simulink model "Noa_Nofusion_angle"  (R2020b)
settings: Solver=FixedStepDiscrete  StartTime=0.0  StopTime=Inf  FixedStep=0.01  RelTol=1e-3
PostLoadFcn:
  | if any(exist('dsrtsu_mdlpostloadfcn', 'file') ~= 0), dsrtsu_mdlpostloadfcn('Execute', bdroot); end
InitFcn:
  | , if any(exist('rtifpga_mdlclblib', 'file') ~= 0), rtifpga_mdlclblib('Init', bdroot); end,
  | , if any(exist('dsmpb_private', 'file') ~= 0), dsmpb_private('dsmpb_mdlclblib', 'Init', bdroot); end,
undefined symbols (not defined in the file): ACC_TimeGap_DecSetSwt, ACC_TimeGap_IncSetSwt, AccelPedalPosn, AccelPedalPosnVldty, AccelPedlPosnDiagc, AccPedalOverride, ACU_ShiftInProgress, ADAS_Posn_CurLane, AESSwtReq, ALC_SwtReq, BrkPedalSts, CC_ACC_CANCEL_OFFSwt, CC_ACC_CRUISE_OFFSwt, CC_ACC_DecSetSpd_SetSwt, CC_ACC_IncSetSpd_ResuSwt, CC_ACCSwtErr, CharSpd_ms, CSA_NODE, CURRENT_GEAR, CurrentGearValid, DiscIntNeverNeededParam, DrvDoorSts, DrvSBR, DrvTrqReqOvld, ECMACCInterface, ECMRespACC, ELKSwtReq, EngLimpHomeSts, EngSpd, EngState, EngState_PHEV, EngTrqMaxActSpd, EngTrqMinAct, EPS_DrvInpTrqVal_HighReslolution, EPS_FailSts, EPS_LKATorqOvrlDlvd, EPS_LKATorqOvrlDlvdVld, EPS_LKATrqOvlDlvdSts, EPS_SteerMod, EPS_TrqSnsrSts, EQ4_APPINFO, EQ4_LA_ELEM, EQ4_LA_HDR, EQ4_LAP_ELEM, EQ4_LAP_HDR, EQ4_LH_ELEM, EQ4_LH_HDR, EQ4_LRE_ELEM, EQ4_LRE_HDR, ESS_PedSwtReq, ESS_VehSwtReq, FFogLmpSts_F_Pbox, FLWheelDriveDirection, FLWheelSpd, FrntWiprSwtSts, FrntWshrSwtSts, FRWheelDriveDirection, FRWheelSpd, HazardLmpSwtSts, HCU_AccelPedalPosn_Diag ... (+151)
libraries: simulink x138, dsmpblib x33, canfdmsglib x10
(part 7 of 17)

== system Noa_Nofusion_angle/EQ4_Lane_Pack1/For Each Subsystem1 ==
  In1 : Inport  Partition=on  PartitionDimension=1  PartitionWidth=1  PartitionOffset=0
  Bus Assignment4 : BusAssignment  AssignedSignals=LH_CRC,LH_Is_Triggered_SDM_Type,LH_Is_Triggered_SDM_Model,LH_Track_ID,LH_Age,LH_Confidence,Reserved_3,LH_Prediction_Reason,LH_Availability_State,LH_Color,LH_Color_Confidence,LH_Lanemark_Type,LH_DLM_Type,LH_DECEL_Type,Reserved_4,LH_Lanemark_Type_Conf,LH_Side,LH_Crossing,LH_Marker_Width,LH_Marker_Width_STD,Reserved_5,LH_Dash_Average_Length,LH_Dash_Average_Gap,LH_Is_Multi_Clothoid,Reserved_6,LH_Line_First_C0,LH_Line_First_C1,LH_Line_First_C2,LH_Line_First_C3,LH_First_VR_Start,LH_First_VR_End,Reserved_7,LH_First_Measured_VR_End,LH_Second_Measured_VR_End,Reserved_8,LH_Line_Second_C0,LH_Line_Second_C1,LH_Line_Second_C2,LH_Line_Second_C3,LH_Second_VR_Start,LH_Second_VR_End,LH_Buffer_C3
  Bus Selector : BusSelector  OutputSignals=LH_CRC,LH_Is_Triggered_SDM_Type,LH_Is_Triggered_SDM_Model,LH_Track_ID,LH_Age,LH_Confidence,Reserved_3,LH_Prediction_Reason,LH_Availability_State,LH_Color,LH_Color_Confidence,LH_Lanemark_Type,LH_DLM_Type,LH_DECEL_Type,Reserved_4,LH_Lanemark_Type_Conf,LH_Side,LH_Crossing,LH_Marker_Width,LH_Marker_Width_STD,Reserved_5,LH_Dash_Average_Length,LH_Dash_Average_Gap,LH_Is_Multi_Clothoid,Reserved_6,LH_Line_First_C0,LH_Line_First_C1,LH_Line_First_C2,LH_Line_First_C3,LH_First_VR_Start,LH_First_VR_End,Reserved_7,LH_First_Measured_VR_End,LH_Second_Measured_VR_End,Reserved_8,LH_Line_Second_C0,LH_Line_Second_C1,LH_Line_Second_C2,LH_Line_Second_C3,LH_Second_VR_Start,LH_Second_VR_End,LH_Buffer_C3
  Constant4 : Constant  Value=0  OutDataTypeStr=Bus: EQ4_LH_ELEM_BUS
  For Each : ForEach  DisableCoverage=on
  Out1 : Outport  ConcatenationDimension=1
  wires:
  Constant4/1 -> Bus Assignment4/1
  In1/1 -> Bus Selector/1
  Bus Assignment4/1 -> Out1/1
  Bus Selector/1 -> Bus Assignment4/2  "<LH_CRC>"
  Bus Selector/2 -> Bus Assignment4/3  "<LH_Is_Triggered_SDM_Type>"
  Bus Selector/3 -> Bus Assignment4/4  "<LH_Is_Triggered_SDM_Model>"
  Bus Selector/4 -> Bus Assignment4/5  "<LH_Track_ID>"
  Bus Selector/5 -> Bus Assignment4/6  "<LH_Age>"
  Bus Selector/6 -> Bus Assignment4/7  "<LH_Confidence>"
  Bus Selector/7 -> Bus Assignment4/8  "<Reserved_3>"
  Bus Selector/8 -> Bus Assignment4/9  "<LH_Prediction_Reason>"
  Bus Selector/9 -> Bus Assignment4/10  "<LH_Availability_State>"
  Bus Selector/10 -> Bus Assignment4/11  "<LH_Color>"
  Bus Selector/11 -> Bus Assignment4/12  "<LH_Color_Confidence>"
  Bus Selector/12 -> Bus Assignment4/13  "<LH_Lanemark_Type>"
  Bus Selector/13 -> Bus Assignment4/14  "<LH_DLM_Type>"
  Bus Selector/14 -> Bus Assignment4/15  "<LH_DECEL_Type>"
  Bus Selector/15 -> Bus Assignment4/16  "<Reserved_4>"
  Bus Selector/16 -> Bus Assignment4/17  "<LH_Lanemark_Type_Conf>"
  Bus Selector/17 -> Bus Assignment4/18  "<LH_Side>"
  Bus Selector/18 -> Bus Assignment4/19  "<LH_Crossing>"
  Bus Selector/19 -> Bus Assignment4/20  "<LH_Marker_Width>"
  Bus Selector/20 -> Bus Assignment4/21  "<LH_Marker_Width_STD>"
  Bus Selector/21 -> Bus Assignment4/22  "<Reserved_5>"
  Bus Selector/22 -> Bus Assignment4/23  "<LH_Dash_Average_Length>"
  Bus Selector/23 -> Bus Assignment4/24  "<LH_Dash_Average_Gap>"
  Bus Selector/24 -> Bus Assignment4/25  "<LH_Is_Multi_Clothoid>"
  Bus Selector/25 -> Bus Assignment4/26  "<Reserved_6>"
  Bus Selector/26 -> Bus Assignment4/27  "<LH_Line_First_C0>"
  Bus Selector/27 -> Bus Assignment4/28  "<LH_Line_First_C1>"
  Bus Selector/28 -> Bus Assignment4/29  "<LH_Line_First_C2>"
  Bus Selector/29 -> Bus Assignment4/30  "<LH_Line_First_C3>"
  Bus Selector/30 -> Bus Assignment4/31  "<LH_First_VR_Start>"
  Bus Selector/31 -> Bus Assignment4/32  "<LH_First_VR_End>"
  Bus Selector/32 -> Bus Assignment4/33  "<Reserved_7>"
  Bus Selector/33 -> Bus Assignment4/34  "<LH_First_Measured_VR_End>"
  Bus Selector/34 -> Bus Assignment4/35  "<LH_Second_Measured_VR_End>"
  Bus Selector/35 -> Bus Assignment4/36  "<Reserved_8>"
  Bus Selector/36 -> Bus Assignment4/37  "<LH_Line_Second_C0>"
  Bus Selector/37 -> Bus Assignment4/38  "<LH_Line_Second_C1>"
  Bus Selector/38 -> Bus Assignment4/39  "<LH_Line_Second_C2>"
  Bus Selector/39 -> Bus Assignment4/40  "<LH_Line_Second_C3>"
  Bus Selector/40 -> Bus Assignment4/41  "<LH_Second_VR_Start>"
  Bus Selector/41 -> Bus Assignment4/42  "<LH_Second_VR_End>"
  Bus Selector/42 -> Bus Assignment4/43  "<LH_Buffer_C3>"

== system Noa_Nofusion_angle/EQ4_Lane_Pack1/For Each Subsystem2 ==
  In1 : Inport  Partition=on  PartitionDimension=1  PartitionWidth=1  PartitionOffset=0
  Bus Assignment4 : BusAssignment  AssignedSignals=LRE_ID,LRE_Age,LRE_Confidence,LRE_Type,Reserved_2,LRE_Prediction_Reason,LRE_Availability_State,LRE_Height,LRE_Height_STD,Reserved_3,LRE_View_Range_Start,LRE_View_Range_End,Reserved_4,LRE_Measured_VR_End,LRE_Side,LRE_Is_Triggered_SDM_Model,Reserved_5,LRE_Line_C3,LRE_Line_C2,LRE_Line_C1,LRE_Line_C0,LRE_Detection_Source,Reserved_6
  Bus Selector : BusSelector  OutputSignals=LRE_ID,LRE_Age,LRE_Confidence,LRE_Type,Reserved_2,LRE_Prediction_Reason,LRE_Availability_State,LRE_Height,LRE_Height_STD,Reserved_3,LRE_View_Range_Start,LRE_View_Range_End,Reserved_4,LRE_Measured_VR_End,LRE_Side,LRE_Is_Triggered_SDM_Model,Reserved_5,LRE_Line_C3,LRE_Line_C2,LRE_Line_C1,LRE_Line_C0,LRE_Detection_Source,Reserved_6
  Constant4 : Constant  Value=0  OutDataTypeStr=Bus: EQ4_LRE_ELEM_BUS
  For Each : ForEach  DisableCoverage=on
  Out1 : Outport  ConcatenationDimension=1
  wires:
  Bus Assignment4/1 -> Out1/1
  In1/1 -> Bus Selector/1
  Constant4/1 -> Bus Assignment4/1
  Bus Selector/1 -> Bus Assignment4/2  "<LRE_ID>"
  Bus Selector/2 -> Bus Assignment4/3  "<LRE_Age>"
  Bus Selector/3 -> Bus Assignment4/4  "<LRE_Confidence>"
  Bus Selector/4 -> Bus Assignment4/5  "<LRE_Type>"
  Bus Selector/5 -> Bus Assignment4/6  "<Reserved_2>"
  Bus Selector/6 -> Bus Assignment4/7  "<LRE_Prediction_Reason>"
  Bus Selector/7 -> Bus Assignment4/8  "<LRE_Availability_State>"
  Bus Selector/8 -> Bus Assignment4/9  "<LRE_Height>"
  Bus Selector/9 -> Bus Assignment4/10  "<LRE_Height_STD>"
  Bus Selector/10 -> Bus Assignment4/11  "<Reserved_3>"
  Bus Selector/11 -> Bus Assignment4/12  "<LRE_View_Range_Start>"
  Bus Selector/12 -> Bus Assignment4/13  "<LRE_View_Range_End>"
  Bus Selector/13 -> Bus Assignment4/14  "<Reserved_4>"
  Bus Selector/14 -> Bus Assignment4/15  "<LRE_Measured_VR_End>"
  Bus Selector/15 -> Bus Assignment4/16  "<LRE_Side>"
  Bus Selector/16 -> Bus Assignment4/17  "<LRE_Is_Triggered_SDM_Model>"
  Bus Selector/17 -> Bus Assignment4/18  "<Reserved_5>"
  Bus Selector/18 -> Bus Assignment4/19  "<LRE_Line_C3>"
  Bus Selector/19 -> Bus Assignment4/20  "<LRE_Line_C2>"
  Bus Selector/20 -> Bus Assignment4/21  "<LRE_Line_C1>"
  Bus Selector/21 -> Bus Assignment4/22  "<LRE_Line_C0>"
  Bus Selector/22 -> Bus Assignment4/23  "<LRE_Detection_Source>"
  Bus Selector/23 -> Bus Assignment4/24  "<Reserved_6>"

== system Noa_Nofusion_angle/EQ4_Lane_Pack1/For Each Subsystem3 ==
  In1 : Inport  Partition=on  PartitionDimension=1  PartitionWidth=1  PartitionOffset=0
  Bus Assignment4 : BusAssignment  AssignedSignals=LA_Lane_Track_ID,LA_Age,LA_Confidence,LA_Color,LA_Color_Conf,LA_Prediction_Reason,LA_Availability_State,LA_View_Range_Start,Reserved_2,LA_View_Range_End,LA_Measured_VR_End,Reserved_3,LA_Lanemark_Type,LA_DLM_Type,LA_Lanemark_Type_Conf,LA_Line_Side,LA_Marker_Width,Reserved_4,LA_Marker_Width_STD,Reserved_5,LA_Line_C3,LA_Line_C2,LA_Line_C1,LA_Line_C0,LH_Buffer_C1,Reserved_6
  Bus Selector : BusSelector  OutputSignals=LA_Lane_Track_ID,LA_Age,LA_Confidence,LA_Color,LA_Color_Conf,LA_Prediction_Reason,LA_Availability_State,LA_View_Range_Start,Reserved_2,LA_View_Range_End,LA_Measured_VR_End,Reserved_3,LA_Lanemark_Type,LA_DLM_Type,LA_Lanemark_Type_Conf,LA_Line_Side,LA_Marker_Width,Reserved_4,LA_Marker_Width_STD,Reserved_5,LA_Line_C3,LA_Line_C2,LA_Line_C1,LA_Line_C0,LH_Buffer_C1,Reserved_6
  Constant4 : Constant  Value=0  OutDataTypeStr=Bus: EQ4_LA_ELEM_BUS
  For Each : ForEach  DisableCoverage=on
  Out1 : Outport  ConcatenationDimension=1
  wires:
  Bus Assignment4/1 -> Out1/1
  In1/1 -> Bus Selector/1
  Constant4/1 -> Bus Assignment4/1
  Bus Selector/1 -> Bus Assignment4/2  "<LA_Lane_Track_ID>"
  Bus Selector/2 -> Bus Assignment4/3  "<LA_Age>"
  Bus Selector/3 -> Bus Assignment4/4  "<LA_Confidence>"
  Bus Selector/4 -> Bus Assignment4/5  "<LA_Color>"
  Bus Selector/5 -> Bus Assignment4/6  "<LA_Color_Conf>"
  Bus Selector/6 -> Bus Assignment4/7  "<LA_Prediction_Reason>"
  Bus Selector/7 -> Bus Assignment4/8  "<LA_Availability_State>"
  Bus Selector/8 -> Bus Assignment4/9  "<LA_View_Range_Start>"
  Bus Selector/9 -> Bus Assignment4/10  "<Reserved_2>"
  Bus Selector/10 -> Bus Assignment4/11  "<LA_View_Range_End>"
  Bus Selector/11 -> Bus Assignment4/12  "<LA_Measured_VR_End>"
  Bus Selector/12 -> Bus Assignment4/13  "<Reserved_3>"
  Bus Selector/13 -> Bus Assignment4/14  "<LA_Lanemark_Type>"
  Bus Selector/14 -> Bus Assignment4/15  "<LA_DLM_Type>"
  Bus Selector/15 -> Bus Assignment4/16  "<LA_Lanemark_Type_Conf>"
  Bus Selector/16 -> Bus Assignment4/17  "<LA_Line_Side>"
  Bus Selector/17 -> Bus Assignment4/18  "<LA_Marker_Width>"
  Bus Selector/18 -> Bus Assignment4/19  "<Reserved_4>"
  Bus Selector/19 -> Bus Assignment4/20  "<LA_Marker_Width_STD>"
  Bus Selector/20 -> Bus Assignment4/21  "<Reserved_5>"
  Bus Selector/21 -> Bus Assignment4/22  "<LA_Line_C3>"
  Bus Selector/22 -> Bus Assignment4/23  "<LA_Line_C2>"
  Bus Selector/23 -> Bus Assignment4/24  "<LA_Line_C1>"
  Bus Selector/24 -> Bus Assignment4/25  "<LA_Line_C0>"
  Bus Selector/25 -> Bus Assignment4/26  "<LH_Buffer_C1>"
  Bus Selector/26 -> Bus Assignment4/27  "<Reserved_6>"

== system Noa_Nofusion_angle/EQ4_Lane_Pack1/For Each Subsystem4 ==
  In1 : Inport  Partition=on  PartitionDimension=1  PartitionWidth=1  PartitionOffset=0
  Bus Assignment4 : BusAssignment  AssignedSignals=LAP_INTP_ID,LAP_INTP_Distance_Age,LAP_INTP_Confidence,LAP_INTP_Is_Valid,LAP_INTP_Type,LAP_INTP_Is_Start,Reserved_4,LAP_INTP_Lat_Distance,LAP_INTP_Long_Distance,Reserved_5,LAP_Buffer_C1,LAP_Buffer_C2,Reserved_6
  Bus Selector : BusSelector  OutputSignals=LAP_INTP_ID,LAP_INTP_Distance_Age,LAP_INTP_Confidence,LAP_INTP_Is_Valid,LAP_INTP_Type,LAP_INTP_Is_Start,Reserved_4,LAP_INTP_Lat_Distance,LAP_INTP_Long_Distance,Reserved_5,LAP_Buffer_C1,LAP_Buffer_C2,Reserved_6,Reserved_7
  Constant4 : Constant  Value=0  OutDataTypeStr=Bus: EQ4_LAP_ELEM_BUS
  For Each : ForEach  DisableCoverage=on
  Out1 : Outport  ConcatenationDimension=1
  wires:
  Constant4/1 -> Bus Assignment4/1
  In1/1 -> Bus Selector/1
  Bus Assignment4/1 -> Out1/1
  Bus Selector/1 -> Bus Assignment4/2  "<LAP_INTP_ID>"
  Bus Selector/2 -> Bus Assignment4/3  "<LAP_INTP_Distance_Age>"
  Bus Selector/3 -> Bus Assignment4/4  "<LAP_INTP_Confidence>"
  Bus Selector/4 -> Bus Assignment4/5  "<LAP_INTP_Is_Valid>"
  Bus Selector/5 -> Bus Assignment4/6  "<LAP_INTP_Type>"
  Bus Selector/6 -> Bus Assignment4/7  "<LAP_INTP_Is_Start>"
  Bus Selector/7 -> Bus Assignment4/8  "<Reserved_4>"
  Bus Selector/8 -> Bus Assignment4/9  "<LAP_INTP_Lat_Distance>"
  Bus Selector/9 -> Bus Assignment4/10  "<LAP_INTP_Long_Distance>"
  Bus Selector/10 -> Bus Assignment4/11  "<Reserved_5>"
  Bus Selector/11 -> Bus Assignment4/12  "<LAP_Buffer_C1>"
  Bus Selector/12 -> Bus Assignment4/13  "<LAP_Buffer_C2>"
  Bus Selector/13 -> Bus Assignment4/14  "<Reserved_6>"

== system Noa_Nofusion_angle/LPV/ABM_Pack ==
  In1 : Inport
  Bus Assignment2 : BusAssignment  AssignedSignals=DrvSBR,PassSBR,VehLgtAccel,VehLatAccel,VehYawRate
  Bus Selector14 : BusSelector  OutputSignals=ABM_NODE.ABM1_MSG.DrvSBR,ABM_NODE.ABM1_MSG.PassSBR,ABM_NODE.ABM2_MSG.VehLgtAccel,ABM_NODE.ABM2_MSG.VehLatAccel,ABM_NODE.ABM2_MSG.VehYawRate
  Constant3 : Constant  Value=0  OutDataTypeStr=Bus: VCAN_ABM_MSG_BUS
  VSM_VCAN_ABM : Outport
  wires:
  Bus Assignment2/1 -> VSM_VCAN_ABM/1
  In1/1 -> Bus Selector14/1
  Constant3/1 -> Bus Assignment2/1
  Bus Selector14/5 -> Bus Assignment2/6  "<VehYawRate>"
  Bus Selector14/4 -> Bus Assignment2/5  "<VehLatAccel>"
  Bus Selector14/3 -> Bus Assignment2/4  "<VehLgtAccel>"
  Bus Selector14/2 -> Bus Assignment2/3  "<PassSBR>"
  Bus Selector14/1 -> Bus Assignment2/2  "<DrvSBR>"

== system Noa_Nofusion_angle/LPV/BCM_Pack ==
  In1 : Inport
  Bus Assignment2 : BusAssignment  AssignedSignals=WiprReq_F_PBOX,DrvDoorSts,PassengerDoorSts,WindshldWiprActvSts,HazardLmpSwtSts,KL30BRelaySts
  Bus Selector10 : BusSelector  OutputSignals=BCM_NODE.BCM8_MSG.WiprReq_F_PBOX,BCM_NODE.BCM1_MSG.DrvDoorSts,BCM_NODE.BCM1_MSG.PassengerDoorSts,BCM_NODE.BCM1_MSG.WindshldWiprActvSts,BCM_NODE.BCM3_MSG.HazardLmpSwtSts,BCM_NODE.BCM8_MSG.KL30BRelaySts
  Constant3 : Constant  Value=0  OutDataTypeStr=Bus: VCAN_BCM_MSG_BUS
  VSM_VCAN_BCM : Outport
  wires:
  In1/1 -> Bus Selector10/1
  Bus Assignment2/1 -> VSM_VCAN_BCM/1
  Constant3/1 -> Bus Assignment2/1
  Bus Selector10/3 -> Bus Assignment2/4  "<PassengerDoorSts>"
  Bus Selector10/4 -> Bus Assignment2/5  "<WindshldWiprActvSts>"
  Bus Selector10/2 -> Bus Assignment2/3  "<DrvDoorSts>"
  Bus Selector10/5 -> Bus Assignment2/6  "<HazardLmpSwtSts>"
  Bus Selector10/1 -> Bus Assignment2/2  "<WiprReq_F_PBOX>"
  Bus Selector10/6 -> Bus Assignment2/7  "<KL30BRelaySts>"

== system Noa_Nofusion_angle/LPV/CSA_Pack ==
  In1 : Inport
  Bus Assignment2 : BusAssignment  AssignedSignals=FrntWshrSwtSts,FrntWiprSwtSts,LTurnLmpSwtSts,RTurnLmpSwtSts,SteerWheelAng,SteerWheelAngSign,SteerWheelSpd,SteerWheelSpdSign,SAS_Sts,ACC_TimeGap_IncSetSwt,ACC_TimeGap_DecSetSwt,CC_ACC_CRUISE_OFFSwt,CC_ACC_CANCEL_OFFSwt,CC_ACC_IncSetSpd_ResuSwt,CC_ACC_DecSetSpd_SetSwt,CC_ACCSwtErr,HWA_OK_OFFSwt
  Bus Selector13 : BusSelector  OutputSignals=CSA_NODE.CSA1_MSG.FrntWshrSwtSts,CSA_NODE.CSA1_MSG.FrntWiprSwtSts,CSA_NODE.CSA1_MSG.LTurnLmpSwtSts,CSA_NODE.CSA1_MSG.RTurnLmpSwtSts,CSA_NODE.CSA2_MSG.SteerWheelAng,CSA_NODE.CSA2_MSG.SteerWheelAngSign,CSA_NODE.CSA2_MSG.SteerWheelSpd,CSA_NODE.CSA2_MSG.SteerWheelSpdSign,CSA_NODE.CSA2_MSG.SAS_Sts,CSA_NODE.CSA2_MSG.ACC_TimeGap_IncSetSwt,CSA_NODE.CSA2_MSG.ACC_TimeGap_DecSetSwt,CSA_NODE.CSA2_MSG.CC_ACC_CRUISE_OFFSwt,CSA_NODE.CSA2_MSG.CC_ACC_CANCEL_OFFSwt,CSA_NODE.CSA2_MSG.CC_ACC_IncSetSpd_ResuSwt,CSA_NODE.CSA2_MSG.CC_ACC_DecSetSpd_SetSwt,CSA_NODE.CSA2_MSG.CC_ACCSwtErr,CSA_NODE.CSA2_MSG.HWA_OK_OFFSwt
  Constant3 : Constant  Value=0  OutDataTypeStr=Bus: VCAN_CSA_MSG_BUS
  VSM_VCAN_CSA : Outport
  wires:
  In1/1 -> Bus Selector13/1
  Bus Assignment2/1 -> VSM_VCAN_CSA/1
  Constant3/1 -> Bus Assignment2/1
  Bus Selector13/1 -> Bus Assignment2/2  "<FrntWshrSwtSts>"
  Bus Selector13/2 -> Bus Assignment2/3  "<FrntWiprSwtSts>"
  Bus Selector13/3 -> Bus Assignment2/4  "<LTurnLmpSwtSts>"
  Bus Selector13/4 -> Bus Assignment2/5  "<RTurnLmpSwtSts>"
  Bus Selector13/5 -> Bus Assignment2/6  "<SteerWheelAng>"
  Bus Selector13/6 -> Bus Assignment2/7  "<SteerWheelAngSign>"
  Bus Selector13/7 -> Bus Assignment2/8  "<SteerWheelSpd>"
  Bus Selector13/8 -> Bus Assignment2/9  "<SteerWheelSpdSign>"
  Bus Selector13/9 -> Bus Assignment2/10  "<SAS_Sts>"
  Bus Selector13/10 -> Bus Assignment2/11  "<ACC_TimeGap_IncSetSwt>"
  Bus Selector13/11 -> Bus Assignment2/12  "<ACC_TimeGap_DecSetSwt>"
  Bus Selector13/12 -> Bus Assignment2/13  "<CC_ACC_CRUISE_OFFSwt>"
  Bus Selector13/13 -> Bus Assignment2/14  "<CC_ACC_CANCEL_OFFSwt>"
  Bus Selector13/14 -> Bus Assignment2/15  "<CC_ACC_IncSetSpd_ResuSwt>"
  Bus Selector13/15 -> Bus Assignment2/16  "<CC_ACC_DecSetSpd_SetSwt>"
  Bus Selector13/16 -> Bus Assignment2/17  "<CC_ACCSwtErr>"
  Bus Selector13/17 -> Bus Assignment2/18  "<HWA_OK_OFFSwt>"

== system Noa_Nofusion_angle/LPV/DCT_Pack ==
  In1 : Inport
  Bus Assignment : BusAssignment  AssignedSignals=CurrentGearValid,SHIFT_IN_PROGRESS,TargetGearValid,TARGET_GEAR,ShiftInPrgValid,CURRENT_GEAR,TGS_LEVER
  Bus Selector7 : BusSelector  OutputSignals=DCT_NODE.DCT5_MSG.CurrentGearValid,DCT_NODE.DCT5_MSG.SHIFT_IN_PROGRESS,DCT_NODE.DCT5_MSG.TargetGearValid,DCT_NODE.DCT5_MSG.TARGET_GEAR,DCT_NODE.DCT5_MSG.ShiftInPrgValid,DCT_NODE.DCT5_MSG.CURRENT_GEAR,DCT_NODE.DCT5_MSG.TGS_LEVER
  Constant1 : Constant  Value=0  OutDataTypeStr=Bus: VCAN_DCT_MSG_BUS
  VSM_VCAN_DCT : Outport
  wires:
  In1/1 -> Bus Selector7/1
  Constant1/1 -> Bus Assignment/1
  Bus Selector7/1 -> Bus Assignment/2  "<CurrentGearValid>"
  Bus Selector7/2 -> Bus Assignment/3  "<SHIFT_IN_PROGRESS>"
  Bus Selector7/3 -> Bus Assignment/4  "<TargetGearValid>"
  Bus Selector7/4 -> Bus Assignment/5  "<TARGET_GEAR>"
  Bus Selector7/5 -> Bus Assignment/6  "<ShiftInPrgValid>"
  Bus Selector7/6 -> Bus Assignment/7  "<CURRENT_GEAR>"
  Bus Selector7/7 -> Bus Assignment/8  "<TGS_LEVER>"
  Bus Assignment/1 -> VSM_VCAN_DCT/1

== system Noa_Nofusion_angle/LPV/ECM_Pack ==
  In1 : Inport
  Bus Assignment : BusAssignment  AssignedSignals=BrkPedalSts,EngSpd,Start_StopSts,AccPedalOverride,AccelPedlPosnDiagc,ECMRespACC,ECMACCInterface,AccelPedalPosn,AccelPedalPosnVldty,EngState,EngLimpHomeSts,EngState_PHEV
  Bus Selector6 : BusSelector  OutputSignals=ECM_NODE.ECM_FD1_MSG.BrkPedalSts,ECM_NODE.ECM_FD1_MSG.EngSpd,ECM_NODE.ECM_FD1_MSG.Start_StopSts,ECM_NODE.ECM_FD2_MSG.AccPedalOverride,ECM_NODE.ECM_FD2_MSG.AccelPedlPosnDiagc,ECM_NODE.ECM_FD2_MSG.ECMRespACC,ECM_NODE.ECM_FD2_MSG.ECMACCInterface,ECM_NODE.ECM_FD2_MSG.AccelPedalPosn,ECM_NODE.ECM_FD2_MSG.AccelPedalPosnVldty,ECM_NODE.ECM_FD2_MSG.EngState,ECM_NODE.ECM_FD3_MSG.EngLimpHomeSts
  Constant : Constant  Value=0x2
  Constant1 : Constant  Value=0  OutDataTypeStr=Bus: VCAN_ECM_MSG_BUS
  VSM_VCAN_ECM : Outport
  wires:
  In1/1 -> Bus Selector6/1
  Constant1/1 -> Bus Assignment/1
  Bus Assignment/1 -> VSM_VCAN_ECM/1
  Bus Selector6/5 -> Bus Assignment/6  "<AccelPedlPosnDiagc>"
  Bus Selector6/4 -> Bus Assignment/5  "<AccPedalOverride>"
  Bus Selector6/6 -> Bus Assignment/7  "<ECMRespACC>"
  Bus Selector6/3 -> Bus Assignment/4  "<Start_StopSts>"
  Bus Selector6/7 -> Bus Assignment/8  "<ECMACCInterface>"
  Bus Selector6/2 -> Bus Assignment/3  "<EngSpd>"
  Bus Selector6/8 -> Bus Assignment/9  "<AccelPedalPosn>"
  Bus Selector6/1 -> Bus Assignment/2  "<BrkPedalSts>"
  Bus Selector6/9 -> Bus Assignment/10  "<AccelPedalPosnVldty>"
  Bus Selector6/10 -> Bus Assignment/11  "<EngState>"
  Bus Selector6/11 -> Bus Assignment/12  "<EngLimpHomeSts>"
  Constant/1 -> Bus Assignment/13

== system Noa_Nofusion_angle/LPV/ESP_Pack ==
  In1 : Inport
  Bus Assignment : BusAssignment  AssignedSignals=BrkDskOvrheatd,NoBrkForce,VehStandstill,HDCCtrl,CDDActv,CDDAvailable,AVHSts,DrivingModDis,ESPFuncOffSts,ESPBrkLmpCtrl,ESPFailSts,ESP_MasterCylBrkPressVld,MSRActv,VDCActv,PTCActv,BTCActv,ESP_MasterCylBrkPress,MSRActv_RA,PTCActv_RA,BTCActv_RA,ABSFailSts,EBDFailSts,VehSpd,ABSActv,EPBSts,EPB_SwtPosn,RLWheelDriveDirection,RLWheelSpd,RRWheelDriveDirection,RRWheelSpd
  Bus Assignment1 : BusAssignment  AssignedSignals=EPS_FailSts,EPS_TrqSnsrSts,EPS_SteerMod,EPS_LKATorqOvrlDlvd,EPS_LKATorqOvrlDlvdVld,EPS_LKATrqOvlDlvdSts,EPS_DrvInpTrqVal_HighReslolution
  Bus Assignment2 : BusAssignment  AssignedSignals=SysPowerMod
  Bus Selector8 : BusSelector  OutputSignals=ESP_NODE.ESP_FD2_MSG.BrkDskOvrheatd,ESP_NODE.ESP_FD2_MSG.NoBrkForce,ESP_NODE.ESP_FD2_MSG.VehStandstill,ESP_NODE.ESP_FD2_MSG.HDCCtrl,ESP_NODE.ESP_FD2_MSG.CDDActv,ESP_NODE.ESP_FD2_MSG.CDDAvailable,ESP_NODE.ESP_FD2_MSG.AVHSts,ESP_NODE.ESP_FD2_MSG.DrivingModDis,ESP_NODE.ESP_FD2_MSG.ESPFuncOffSts,ESP_NODE.ESP_FD2_MSG.ESPBrkLmpCtrl,ESP_NODE.ESP_FD2_MSG.ESPFailSts,ESP_NODE.ESP_FD2_MSG.ESP_MasterCylBrkPressVld,ESP_NODE.ESP_FD2_MSG.MSRActv,ESP_NODE.ESP_FD2_MSG.VDCActv,ESP_NODE.ESP_FD2_MSG.PTCActv,ESP_NODE.ESP_FD2_MSG.BTCActv,ESP_NODE.ESP_FD2_MSG.ESP_MasterCylBrkPress,ESP_NODE.ESP_FD2_MSG.MSRActv_RA,ESP_NODE.ESP_FD2_MSG.PTCActv_RA,ESP_NODE.ESP_FD2_MSG.BTCActv_RA,ESP_NODE.ESP_FD2_MSG.ABSFailSts,ESP_NODE.ESP_FD2_MSG.EBDFailSts,ESP_NODE.ESP_FD2_MSG.VehSpd,ESP_NODE.ESP_FD2_MSG.ABSActv,ESP_NODE.ESP_FD3_MSG.EPBSts,ESP_NODE.ESP_FD3_MSG.EPB_SwtPosn,ESP_NODE.ESP_FD3_MSG.RLWheelDriveDirection,ESP_NODE.ESP_FD3_MSG.RLWheelSpd,ESP_NODE.ESP_FD3_MSG.RRWheelDriveDirection,ESP_NODE.ESP_FD3_MSG.RRWheelSpd,EPS_NODE.EPS_FD1_MSG.EPS_FailSts,EPS_NODE.EPS_FD1_MSG.EPS_TrqSnsrSts,EPS_NODE.EPS_FD1_MSG.EPS_SteerMod,EPS_NODE.EPS_FD1_MSG.EPS_LKATorqOvrlDlvd,EPS_NODE.EPS_FD1_MSG.EPS_LKATorqOvrlDlvdVld,EPS_NODE.EPS_FD1_MSG.EPS_LKATrqOvlDlvdSts,EPS_NODE.EPS_FD1_MSG.EPS_DrvInpTrqVal_HighReslolution,PEPS_NODE.PEPS2_MSG.SysPowerMod
  Constant1 : Constant  Value=0  OutDataTypeStr=Bus: VCAN_ESP_MSG_BUS
  Constant2 : Constant  Value=0  OutDataTypeStr=Bus: VCAN_EPS_MSG_BUS
  Constant3 : Constant  Value=0  OutDataTypeStr=Bus: VCAN_PEPS_MSG_BUS
  VSM_VCAN_ESP : Outport
  VSM_VCAN_EPS : Outport  Port=2
  VSM_VCAN_PEPS : Outport  Port=3
  wires:
  In1/1 -> Bus Selector8/1
  Constant1/1 -> Bus Assignment/1
  Bus Selector8/6 -> Bus Assignment/7  "<CDDAvailable>"
  Bus Selector8/7 -> Bus Assignment/8  "<AVHSts>"
  Bus Selector8/5 -> Bus Assignment/6  "<CDDActv>"
  Bus Selector8/8 -> Bus Assignment/9  "<DrivingModDis>"
  Bus Selector8/4 -> Bus Assignment/5  "<HDCCtrl>"
  Bus Selector8/9 -> Bus Assignment/10  "<ESPFuncOffSts>"
  Bus Selector8/3 -> Bus Assignment/4  "<VehStandstill>"
  Bus Selector8/10 -> Bus Assignment/11  "<ESPBrkLmpCtrl>"
  Bus Selector8/2 -> Bus Assignment/3  "<NoBrkForce>"
  Bus Selector8/11 -> Bus Assignment/12  "<ESPFailSts>"
  Bus Selector8/1 -> Bus Assignment/2  "<BrkDskOvrheatd>"
  Bus Selector8/12 -> Bus Assignment/13  "<ESP_MasterCylBrkPressVld>"
  Bus Selector8/13 -> Bus Assignment/14  "<MSRActv>"
  Bus Selector8/14 -> Bus Assignment/15  "<VDCActv>"
  Bus Selector8/15 -> Bus Assignment/16  "<PTCActv>"
  Bus Selector8/16 -> Bus Assignment/17  "<BTCActv>"
  Bus Selector8/17 -> Bus Assignment/18  "<ESP_MasterCylBrkPress>"
  Bus Selector8/18 -> Bus Assignment/19  "<MSRActv_RA>"
  Bus Selector8/19 -> Bus Assignment/20  "<PTCActv_RA>"
  Bus Selector8/20 -> Bus Assignment/21  "<BTCActv_RA>"
  Bus Selector8/21 -> Bus Assignment/22  "<ABSFailSts>"
  Bus Selector8/22 -> Bus Assignment/23  "<EBDFailSts>"
  Bus Selector8/23 -> Bus Assignment/24  "<VehSpd>"
  Bus Selector8/24 -> Bus Assignment/25  "<ABSActv>"
  Bus Selector8/25 -> Bus Assignment/26  "<EPBSts>"
  Bus Selector8/26 -> Bus Assignment/27  "<EPB_SwtPosn>"
  Bus Selector8/27 -> Bus Assignment/28  "<RLWheelDriveDirection>"
  Bus Selector8/28 -> Bus Assignment/29  "<RLWheelSpd>"
  Bus Selector8/29 -> Bus Assignment/30  "<RRWheelDriveDirection>"
  Bus Selector8/30 -> Bus Assignment/31  "<RRWheelSpd>"
  Bus Assignment/1 -> VSM_VCAN_ESP/1
  Constant2/1 -> Bus Assignment1/1
  Bus Selector8/33 -> Bus Assignment1/4  "<EPS_SteerMod>"
  Bus Selector8/34 -> Bus Assignment1/5  "<EPS_LKATorqOvrlDlvd>"
  Bus Selector8/32 -> Bus Assignment1/3  "<EPS_TrqSnsrSts>"
  Bus Selector8/35 -> Bus Assignment1/6  "<EPS_LKATorqOvrlDlvdVld>"
  Bus Selector8/31 -> Bus Assignment1/2  "<EPS_FailSts>"
  Bus Selector8/36 -> Bus Assignment1/7  "<EPS_LKATrqOvlDlvdSts>"
  Bus Selector8/37 -> Bus Assignment1/8  "<EPS_DrvInpTrqVal_HighReslolution>"
  Bus Selector8/38 -> Bus Assignment2/2  "<SysPowerMod>"
  Constant3/1 -> Bus Assignment2/1
  Bus Assignment1/1 -> VSM_VCAN_EPS/1
  Bus Assignment2/1 -> VSM_VCAN_PEPS/1

== system Noa_Nofusion_angle/LPV/HAP_Pack ==
  In1 : Inport
  Bus Assignment2 : BusAssignment  AssignedSignals=USS_FrontSys_Status,USS_FLCNear_Obj_Confidence,USS_FLCNear_Obj_Pos_X,USS_FLCNear_Obj_Pos_Y,USS_FLMNear_Obj_Confidence,USS_FLMNear_Obj_Pos_X,USS_FLMNear_Obj_Pos_Y,USS_FRMNear_Obj_Confidence,USS_FRMNear_Obj_Pos_X,USS_FRMNear_Obj_Pos_Y,USS_FRCNear_Obj_Confidence,USS_FRCNear_Obj_Pos_X,USS_FRCNear_Obj_Pos_Y,APS_WorkSts,DVRWorkSts
  Bus Selector18 : BusSelector  OutputSignals=HAP_NODE.HAP_FD6_MSG.USS_FrontSys_Status,HAP_NODE.HAP_FD6_MSG.USS_FLCNear_Obj_Confidence,HAP_NODE.HAP_FD6_MSG.USS_FLCNear_Obj_Pos_X,HAP_NODE.HAP_FD6_MSG.USS_FLCNear_Obj_Pos_Y,HAP_NODE.HAP_FD6_MSG.USS_FLMNear_Obj_Confidence,HAP_NODE.HAP_FD6_MSG.USS_FLMNear_Obj_Pos_X,HAP_NODE.HAP_FD6_MSG.USS_FLMNear_Obj_Pos_Y,HAP_NODE.HAP_FD6_MSG.USS_FRMNear_Obj_Confidence,HAP_NODE.HAP_FD6_MSG.USS_FRMNear_Obj_Pos_X,HAP_NODE.HAP_FD6_MSG.USS_FRMNear_Obj_Pos_Y,HAP_NODE.HAP_FD6_MSG.USS_FRCNear_Obj_Confidence,HAP_NODE.HAP_FD6_MSG.USS_FRCNear_Obj_Pos_X,HAP_NODE.HAP_FD6_MSG.USS_FRCNear_Obj_Pos_Y,HAP_NODE.HAP_FD1_MSG.APS_WorkSts,HAP_NODE.HAP_FD2_MSG.DVRWorkSts
  Constant3 : Constant  Value=0  OutDataTypeStr=Bus: VCAN_HAP_MSG_BUS
  VSM_VCAN_HAP : Outport
  wires:
  In1/1 -> Bus Selector18/1
  Constant3/1 -> Bus Assignment2/1
  Bus Selector18/1 -> Bus Assignment2/2  "<USS_FrontSys_Status>"
  Bus Selector18/2 -> Bus Assignment2/3  "<USS_FLCNear_Obj_Confidence>"
  Bus Selector18/3 -> Bus Assignment2/4  "<USS_FLCNear_Obj_Pos_X>"
  Bus Selector18/4 -> Bus Assignment2/5  "<USS_FLCNear_Obj_Pos_Y>"
  Bus Selector18/5 -> Bus Assignment2/6  "<USS_FLMNear_Obj_Confidence>"
  Bus Selector18/6 -> Bus Assignment2/7  "<USS_FLMNear_Obj_Pos_X>"
  Bus Selector18/7 -> Bus Assignment2/8  "<USS_FLMNear_Obj_Pos_Y>"
  Bus Selector18/8 -> Bus Assignment2/9  "<USS_FRMNear_Obj_Confidence>"
  Bus Selector18/9 -> Bus Assignment2/10  "<USS_FRMNear_Obj_Pos_X>"
  Bus Selector18/10 -> Bus Assignment2/11  "<USS_FRMNear_Obj_Pos_Y>"
  Bus Selector18/11 -> Bus Assignment2/12  "<USS_FRCNear_Obj_Confidence>"
  Bus Selector18/12 -> Bus Assignment2/13  "<USS_FRCNear_Obj_Pos_X>"
  Bus Selector18/13 -> Bus Assignment2/14  "<USS_FRCNear_Obj_Pos_Y>"
  Bus Selector18/14 -> Bus Assignment2/15  "<APS_WorkSts>"
  Bus Selector18/15 -> Bus Assignment2/16  "<DVRWorkSts>"
  Bus Assignment2/1 -> VSM_VCAN_HAP/1

== system Noa_Nofusion_angle/LPV/HUT_Pack ==
  In1 : Inport
  Bus Assignment1 : BusAssignment  AssignedSignals=CR_BrkgReq
  Bus Assignment2 : BusAssignment  AssignedSignals=IFC_SnvtySet,LKASwtReq,LCKSwtReq,ELKSwtReq,ESS_PedSwtReq,ESS_VehSwtReq,LDWSwtReq,TSRSwtReq,TSRWarnSwtReq,ICA_HandsOffSwtReq,ISLSwtReq,TSR_SnvtySet,LSSWarnFormSwtReq,LSSSwtReq,IntelligentEvaSwtReq,AESSwtReq,HWA_SwtReq,HWA_SnvtySet,ALC_SwtReq
  Bus Selector16 : BusSelector  OutputSignals=HUT_NODE.HUT_FD1_MSG.IFC_SnvtySet,HUT_NODE.HUT_FD1_MSG.LKASwtReq,HUT_NODE.HUT_FD1_MSG.LCKSwtReq,HUT_NODE.HUT_FD1_MSG.ELKSwtReq,HUT_NODE.HUT_FD1_MSG.ESS_PedSwtReq,HUT_NODE.HUT_FD1_MSG.ESS_VehSwtReq,HUT_NODE.HUT_FD1_MSG.LDWSwtReq,HUT_NODE.HUT_FD1_MSG.TSRSwtReq,HUT_NODE.HUT_FD1_MSG.TSRWarnSwtReq,HUT_NODE.HUT_FD1_MSG.ICA_HandsOffSwtReq,HUT_NODE.HUT_FD1_MSG.ISLSwtReq,HUT_NODE.HUT_FD1_MSG.TSR_SnvtySet,HUT_NODE.HUT_FD1_MSG.LSSWarnFormSwtReq,HUT_NODE.HUT_FD1_MSG.LSSSwtReq,HUT_NODE.HUT_FD1_MSG.IntelligentEvaSwtReq,HUT_NODE.HUT_FD1_MSG.AESSwtReq,HUT_NODE.HUT_FD1_MSG.HWA_SwtReq,HUT_NODE.HUT_FD1_MSG.HWA_SnvtySet,HUT_NODE.HUT_FD1_MSG.ALC_SwtReq,CR_NODE.CR_FD1_MSG.CR_BrkgReq
  Constant1 : Constant  Value=0  OutDataTypeStr=Bus: VCAN_CR_MSG_BUS
  Constant3 : Constant  Value=0  OutDataTypeStr=Bus: VCAN_HUT_MSG_BUS
  VSM_VCAN_HUT : Outport
  VSM_VCAN_CR : Outport  Port=2
  wires:
  In1/1 -> Bus Selector16/1
  Constant3/1 -> Bus Assignment2/1
  Bus Selector16/1 -> Bus Assignment2/2  "<IFC_SnvtySet>"
  Bus Selector16/2 -> Bus Assignment2/3  "<LKASwtReq>"
  Bus Selector16/3 -> Bus Assignment2/4  "<LCKSwtReq>"
  Bus Selector16/4 -> Bus Assignment2/5  "<ELKSwtReq>"
  Bus Selector16/5 -> Bus Assignment2/6  "<ESS_PedSwtReq>"
  Bus Selector16/6 -> Bus Assignment2/7  "<ESS_VehSwtReq>"
  Bus Selector16/7 -> Bus Assignment2/8  "<LDWSwtReq>"
  Bus Selector16/8 -> Bus Assignment2/9  "<TSRSwtReq>"
  Bus Selector16/9 -> Bus Assignment2/10  "<TSRWarnSwtReq>"
  Bus Selector16/10 -> Bus Assignment2/11  "<ICA_HandsOffSwtReq>"
  Bus Selector16/11 -> Bus Assignment2/12  "<ISLSwtReq>"
  Bus Selector16/12 -> Bus Assignment2/13  "<TSR_SnvtySet>"
  Bus Selector16/13 -> Bus Assignment2/14  "<LSSWarnFormSwtReq>"
  Bus Selector16/14 -> Bus Assignment2/15  "<LSSSwtReq>"
  Bus Selector16/15 -> Bus Assignment2/16  "<IntelligentEvaSwtReq>"
  Bus Selector16/16 -> Bus Assignment2/17  "<AESSwtReq>"
  Bus Selector16/17 -> Bus Assignment2/18  "<HWA_SwtReq>"
  Bus Selector16/18 -> Bus Assignment2/19  "<HWA_SnvtySet>"
  Bus Selector16/19 -> Bus Assignment2/20  "<ALC_SwtReq>"
  Bus Assignment2/1 -> VSM_VCAN_HUT/1
  Constant1/1 -> Bus Assignment1/1
  Bus Selector16/20 -> Bus Assignment1/2  "<CR_BrkgReq>"
  Bus Assignment1/1 -> VSM_VCAN_CR/1

== system Noa_Nofusion_angle/LPV/Subsystem ==
  In1 : Inport
  Bus Assignment2 : BusAssignment  AssignedSignals=ACAmbTemp
  Bus Selector11 : BusSelector  OutputSignals=AC_NEDE.AC2_MSG.ACAmbTemp
  Constant3 : Constant  Value=0  OutDataTypeStr=Bus: VCAN_AC_MSG_BUS
  <ACAmbTemp> : Outport
  wires:
  In1/1 -> Bus Selector11/1
  Bus Selector11/1 -> Bus Assignment2/2  "<ACAmbTemp>"
  Constant3/1 -> Bus Assignment2/1
  Bus Assignment2/1 -> <ACAmbTemp>/1

== system Noa_Nofusion_angle/LPV/Subsystem1 ==
  In1 : Inport
  Bus Assignment2 : BusAssignment  AssignedSignals=IP_VehSpdUnit
  Bus Selector15 : BusSelector  OutputSignals=IP_NODE.IP2_MSG.IP_VehSpdUnit
  Constant3 : Constant  Value=0  OutDataTypeStr=Bus: VCAN_IP_MSG_BUS
  <IP_VehSpdUnit> : Outport
  wires:
  In1/1 -> Bus Selector15/1
  Constant3/1 -> Bus Assignment2/1
  Bus Selector15/1 -> Bus Assignment2/2  "<IP_VehSpdUnit>"
  Bus Assignment2/1 -> <IP_VehSpdUnit>/1

== system Noa_Nofusion_angle/LPV/Subsystem2 ==
  In1 : Inport
  Bus Assignment2 : BusAssignment  AssignedSignals=HighBeamSts_HC
  Bus Selector17 : BusSelector  OutputSignals=HC_NODE.HC1_MSG.HighBeamSts_HC
  Constant3 : Constant  Value=0  OutDataTypeStr=Bus: VCAN_HC_MSG_BUS
  <HighBeamSts_HC> : Outport
  wires:
  In1/1 -> Bus Selector17/1
  Constant3/1 -> Bus Assignment2/1
  Bus Selector17/1 -> Bus Assignment2/2  "<HighBeamSts_HC>"
  Bus Assignment2/1 -> <HighBeamSts_HC>/1

== system Noa_Nofusion_angle/LPV/Subsystem3 ==
  In1 : Inport
  Bus Assignment2 : BusAssignment  AssignedSignals=HoodSts_F_Pbox,FFogLmpSts_F_Pbox,RFogLmpSts_R_Pbox,LowBeamSts_F_Pbox
  Bus Selector12 : BusSelector  OutputSignals=PBOX_NODE.F_PBOX1_MSG.HoodSts_F_Pbox,PBOX_NODE.F_PBOX1_MSG.FFogLmpSts_F_Pbox,PBOX_NODE.R_PBOX1_MSG.RFogLmpSts_R_Pbox,PBOX_NODE.F_PBOX1_MSG.LowBeamSts_F_Pbox
  Constant3 : Constant  Value=0  OutDataTypeStr=Bus: VCAN_PBOX_MSG_BUS
  VSM_VCAN_PBOX : Outport
  wires:
  Bus Assignment2/1 -> VSM_VCAN_PBOX/1
  In1/1 -> Bus Selector12/1
  Constant3/1 -> Bus Assignment2/1
  Bus Selector12/4 -> Bus Assignment2/5  "<LowBeamSts_F_Pbox>"
  Bus Selector12/3 -> Bus Assignment2/4  "<RFogLmpSts_R_Pbox>"
  Bus Selector12/2 -> Bus Assignment2/3  "<FFogLmpSts_F_Pbox>"
  Bus Selector12/1 -> Bus Assignment2/2  "<HoodSts_F_Pbox>"

== system Noa_Nofusion_angle/LPV/Subsystem4 ==
  In1 : Inport
  Bus Assignment4 : BusAssignment  AssignedSignals=HCU_BrkPedalSts,HCU_AccelPedalPosn_Diag,HCU_ACCInterface,HCU_PowertrainSts,ACU_ShiftInProgress,HCU_DrvMod,HCU_PTDrvMod,DrvTrqReqOvld,HCU_GearSts
  Bus Selector11 : BusSelector  OutputSignals=HCU_NODE.HCU_FD1_MSG.HCU_BrkPedalSts,HCU_NODE.HCU_FD1_MSG.HCU_AccelPedalPosn_Diag,HCU_NODE.HCU_FD1_MSG.HCU_ACCInterface,HCU_NODE.HCU_FD1_MSG.HCU_PowertrainSts,HCU_NODE.HCU_FD1_MSG.ACU_ShiftInProgress,HCU_NODE.HCU_FD3_MSG.HCU_DrvMod,HCU_NODE.HCU_FD3_MSG.HCU_PTDrvMod,HCU_NODE.HCU_FD3_MSG.DrvTrqReqOvld,HCU_NODE.HCU_FD3_MSG.HCU_GearSts
  Constant4 : Constant  Value=0  OutDataTypeStr=Bus: VCAN_HCU_MSG_BUS
  Out1 : Outport
  wires:
  Bus Selector11/4 -> Bus Assignment4/5  "<HCU_PowertrainSts>"
  Bus Selector11/6 -> Bus Assignment4/7  "<HCU_DrvMod>"
  Constant4/1 -> Bus Assignment4/1
  Bus Selector11/1 -> Bus Assignment4/2  "<HCU_BrkPedalSts>"
  Bus Selector11/8 -> Bus Assignment4/9  "<DrvTrqReqOvld>"
  Bus Selector11/5 -> Bus Assignment4/6  "<ACU_ShiftInProgress>"
  Bus Selector11/2 -> Bus Assignment4/3  "<HCU_AccelPedalPosn_Diag>"
  Bus Assignment4/1 -> Out1/1
  Bus Selector11/3 -> Bus Assignment4/4  "<HCU_ACCInterface>"
  Bus Selector11/7 -> Bus Assignment4/8  "<HCU_PTDrvMod>"
  Bus Selector11/9 -> Bus Assignment4/10  "<HCU_GearSts>"
  In1/1 -> Bus Selector11/1

== system Noa_Nofusion_angle/LPV/Subsystem5 ==
  TOS_P0_TARGET_LINE : Inport  OutDataTypeStr=Bus: TOS_P0_TARGET_LINE_BUS  PortDimensions=1  BusOutputAsStruct=on
  VSM_HMI : Inport  Port=2  OutDataTypeStr=Bus: VSM_HMI_BUS  PortDimensions=1  BusOutputAsStruct=on
  VSM_ReqMRC : Inport  Port=3  OutDataTypeStr=uint8
  vxvRefMs : Inport  Port=4  OutDataTypeStr=single  PortDimensions=1  BusOutputAsStruct=on
  kapTraj : Inport  Port=5  OutDataTypeStr=single  PortDimensions=1  BusOutputAsStruct=on
  PLAN_ALC_DECS : Inport  Port=6  OutDataTypeStr=Bus: PLAN_ALC_DECS_BUS  PortDimensions=1  BusOutputAsStruct=on
  RFM_ROAD : Inport  Port=7  OutDataTypeStr=Bus: RFM_ROAD_BUS  PortDimensions=1  BusOutputAsStruct=on
  RFM_UpdateCnt : Inport  Port=8  OutDataTypeStr=uint32  PortDimensions=1  BusOutputAsStruct=on
  RFM_BRANCH_LANE : Inport  Port=9  OutDataTypeStr=Bus: RFM_LANE_BUS  PortDimensions=1  BusOutputAsStruct=on
  RFM_LEFT_LANE : Inport  Port=10  OutDataTypeStr=Bus: RFM_LANE_BUS  PortDimensions=1  BusOutputAsStruct=on
  RFM_CURRENT_LANE : Inport  Port=11  OutDataTypeStr=Bus: RFM_LANE_BUS  PortDimensions=1  BusOutputAsStruct=on
  RFM_RIGHT_LANE : Inport  Port=12  OutDataTypeStr=Bus: RFM_LANE_BUS  PortDimensions=1  BusOutputAsStruct=on
  RFM_INTERSEC_ALERT : Inport  Port=13  OutDataTypeStr=Bus: RFM_INTERSEC_ALERT_BUS  PortDimensions=1  BusOutputAsStruct=on
  RFM_BRANCH : Inport  Port=14  OutDataTypeStr=Bus: RFM_BRANCH_BUS  PortDimensions=1  BusOutputAsStruct=on
  RFM_REC_LANES : Inport  Port=15  OutDataTypeStr=Bus: RFM_REC_LANES_BUS  PortDimensions=1  BusOutputAsStruct=on
  RFM_LINE_L1 : Inport  Port=16  OutDataTypeStr=Bus: RFM_LINE_BUS  PortDimensions=1  BusOutputAsStruct=on
  RFM_LINE_R1 : Inport  Port=17  OutDataTypeStr=Bus: RFM_LINE_BUS  PortDimensions=1  BusOutputAsStruct=on
  RFM_LINE_L2 : Inport  Port=18  OutDataTypeStr=Bus: RFM_LINE_BUS  PortDimensions=1  BusOutputAsStruct=on
  RFM_LINE_R2 : Inport  Port=19  OutDataTypeStr=Bus: RFM_LINE_BUS  PortDimensions=1  BusOutputAsStruct=on
  RFM_LINE_L3 : Inport  Port=20  OutDataTypeStr=Bus: RFM_LINE_BUS  PortDimensions=1  BusOutputAsStruct=on
  RFM_LINE_R3 : Inport  Port=21  OutDataTypeStr=Bus: RFM_LINE_BUS  PortDimensions=1  BusOutputAsStruct=on
  RFM_LINE_CL : Inport  Port=22  OutDataTypeStr=Bus: RFM_LINE_BUS  PortDimensions=1  BusOutputAsStruct=on
  RFM_LINE_LB : Inport  Port=23  OutDataTypeStr=Bus: RFM_LINE_BUS  PortDimensions=1  BusOutputAsStruct=on
  RFM_LINE_RB : Inport  Port=24  OutDataTypeStr=Bus: RFM_LINE_BUS  PortDimensions=1  BusOutputAsStruct=on
  RFM_LINE_PRED : Inport  Port=25  OutDataTypeStr=Bus: RFM_LINE_BUS  PortDimensions=1  BusOutputAsStruct=on
  RFM_LINEF_LB : Inport  Port=26  OutDataTypeStr=Bus: RFM_LINE_BUS  PortDimensions=1  BusOutputAsStruct=on
  RFM_LINEF_RB : Inport  Port=27  OutDataTypeStr=Bus: RFM_LINE_BUS  PortDimensions=1  BusOutputAsStruct=on
  RFM_LINE_ENTRY_CL : Inport  Port=28  OutDataTypeStr=Bus: RFM_LINE_BUS  PortDimensions=1  BusOutputAsStruct=on
  RFM_LINE_EXIT_CL : Inport  Port=29  OutDataTypeStr=Bus: RFM_LINE_BUS  PortDimensions=1  BusOutputAsStruct=on
  EQ4_LH_HDR : Inport  Port=30  OutDataTypeStr=Bus: EQ4_LH_HDR_BUS  PortDimensions=1  BusOutputAsStruct=on
  EQ4_LH_ELEM : Inport  Port=31  OutDataTypeStr=Bus: EQ4_LH_ELEM_BUS  PortDimensions=1  BusOutputAsStruct=on
  EQ4_LH_ELEM1 : Inport  Port=32  OutDataTypeStr=Bus: EQ4_LH_ELEM_BUS  PortDimensions=1  BusOutputAsStruct=on
  EQ4_LA_HDR : Inport  Port=33  OutDataTypeStr=Bus: EQ4_LA_HDR_BUS  PortDimensions=1  BusOutputAsStruct=on
  EQ4_LA_ELEM : Inport  Port=34  OutDataTypeStr=Bus: EQ4_LA_ELEM_BUS  PortDimensions=1  BusOutputAsStruct=on
  EQ4_LA_ELEM1 : Inport  Port=35  OutDataTypeStr=Bus: EQ4_LA_ELEM_BUS  PortDimensions=1  BusOutputAsStruct=on
  EQ4_LA_ELEM2 : Inport  Port=36  OutDataTypeStr=Bus: EQ4_LA_ELEM_BUS  PortDimensions=1  BusOutputAsStruct=on
  EQ4_LA_ELEM3 : Inport  Port=37  OutDataTypeStr=Bus: EQ4_LA_ELEM_BUS  PortDimensions=1  BusOutputAsStruct=on
  EQ4_LRE_HDR : Inport  Port=38  OutDataTypeStr=Bus: EQ4_LRE_HDR_BUS  PortDimensions=1  BusOutputAsStruct=on
  EQ4_LRE_ELEM : Inport  Port=39  OutDataTypeStr=Bus: EQ4_LRE_ELEM_BUS  PortDimensions=1  BusOutputAsStruct=on
  EQ4_LRE_ELEM1 : Inport  Port=40  OutDataTypeStr=Bus: EQ4_LRE_ELEM_BUS  PortDimensions=1  BusOutputAsStruct=on
  RFM_TSR : Inport  Port=41  OutDataTypeStr=Bus: RFM_TSR_BUS  PortDimensions=1  BusOutputAsStruct=on
  Bus Assignment1 : BusAssignment  AssignedSignals=EQ4_LH_HDR,EQ4_LH_ELEM
  Bus Assignment2 : BusAssignment  AssignedSignals=EQ4_LRE_HDR,EQ4_LRE_ELEM
  Bus Assignment3 : BusAssignment  AssignedSignals=EQ4_LA_HDR,EQ4_LA_ELEM
  Constant1 : Constant  Value=0  OutDataTypeStr=Bus: EQ4_LA_BUS
  Constant2 : Constant  Value=0  OutDataTypeStr=Bus: EQ4_LH_BUS
  Constant3 : Constant  Value=0  OutDataTypeStr=Bus: EQ4_LRE_BUS
  For Each Subsystem1 : Subsystem  TreatAsAtomicUnit=on
  For Each Subsystem2 : Subsystem  TreatAsAtomicUnit=on
  For Each Subsystem3 : Subsystem  TreatAsAtomicUnit=on
  LSM : ModelReference  ModelNameDialog=PubIfDecisionLSM_MDL.slx  SimulationMode=Normal  ModelReferenceVersion=1.510
  Matrix Concatenate : Concatenate  Mode=Multidimensional array
  Matrix Concatenate1 : Concatenate  NumInputs=4  Mode=Multidimensional array
  Matrix Concatenate2 : Concatenate  Mode=Multidimensional array
  Terminator : Terminator
  LSM_TJA_ICA : Outport  OutDataTypeStr=Bus: LSM_TJA_ICA_BUS  PortDimensions=1  BusOutputAsStruct=on
  LSM_LCK : Outport  Port=2  OutDataTypeStr=Bus: LSM_LCK_BUS  PortDimensions=1  BusOutputAsStruct=on
  LSM_HWA : Outport  Port=3  OutDataTypeStr=Bus: LSM_HWA_BUS  PortDimensions=1  BusOutputAsStruct=on
  LSM_ESS : Outport  Port=4  OutDataTypeStr=Bus: LSM_ESS_BUS  PortDimensions=1  BusOutputAsStruct=on
  LSM_UpdateCnt : Outport  Port=5  OutDataTypeStr=uint32  PortDimensions=1  BusOutputAsStruct=on
  LSM_PilotTurnSwSts : Outport  Port=6  OutDataTypeStr=uint8  PortDimensions=1  BusOutputAsStruct=on
  LSM_PilotSts : Outport  Port=7  OutDataTypeStr=uint8  PortDimensions=1  BusOutputAsStruct=on
  LSM_PilotNohExitDist : Outport  Port=8  OutDataTypeStr=uint16  PortDimensions=1  BusOutputAsStruct=on
  LSM_PilotSPLDist : Outport  Port=9  OutDataTypeStr=uint16  PortDimensions=1  BusOutputAsStruct=on
  LSM_PilotSPL : Outport  Port=10  OutDataTypeStr=uint8  PortDimensions=1  BusOutputAsStruct=on
  LSM_PilotRoadSts : Outport  Port=11  OutDataTypeStr=uint8  PortDimensions=1  BusOutputAsStruct=on
  LSM_TJALineSource : Outport  Port=12
  wires:
  For Each Subsystem1/1(Out1) -> Bus Assignment1/3
  For Each Subsystem2/1(Out1) -> Bus Assignment2/3
  LSM/5 -> LSM_UpdateCnt/1
  EQ4_LH_HDR/1 -> Bus Assignment1/2
  Matrix Concatenate/1 -> For Each Subsystem1/1(In1)
  EQ4_LA_ELEM1/1 -> Matrix Concatenate1/2
  Constant3/1 -> Bus Assignment2/1
  For Each Subsystem3/1(Out1) -> Bus Assignment3/3
  LSM/1 -> LSM_TJA_ICA/1
  LSM/11 -> LSM_PilotRoadSts/1
  LSM/8 -> LSM_PilotNohExitDist/1
  Bus Assignment2/1 -> LSM/4
  LSM/3 -> LSM_HWA/1
  LSM/9 -> LSM_PilotSPLDist/1
  EQ4_LH_ELEM1/1 -> Matrix Concatenate/2
  EQ4_LA_ELEM2/1 -> Matrix Concatenate1/3
  LSM/4 -> LSM_ESS/1
  Bus Assignment3/1 -> LSM/3
  EQ4_LRE_HDR/1 -> Bus Assignment2/2
  TOS_P0_TARGET_LINE/1 -> LSM/5
  EQ4_LRE_ELEM1/1 -> Matrix Concatenate2/2
  LSM/7 -> LSM_PilotSts/1
  Matrix Concatenate2/1 -> For Each Subsystem2/1(In1)
  VSM_HMI/1 -> LSM/6
  LSM/2 -> LSM_LCK/1
  LSM/6 -> LSM_PilotTurnSwSts/1
  Bus Assignment1/1 -> LSM/2
  EQ4_LH_ELEM/1 -> Matrix Concatenate/1
  Constant1/1 -> Bus Assignment3/1
  Constant2/1 -> Bus Assignment1/1
  EQ4_LA_ELEM3/1 -> Matrix Concatenate1/4
  EQ4_LRE_ELEM/1 -> Matrix Concatenate2/1
  EQ4_LA_ELEM/1 -> Matrix Concatenate1/1
  Matrix Concatenate1/1 -> For Each Subsystem3/1(In1)
  EQ4_LA_HDR/1 -> Bus Assignment3/2
  LSM/10 -> LSM_PilotSPL/1
  vxvRefMs/1 -> LSM/7
  kapTraj/1 -> LSM/8
  PLAN_ALC_DECS/1 -> LSM/9
  RFM_ROAD/1 -> LSM/10
  RFM_UpdateCnt/1 -> LSM/11
  RFM_BRANCH_LANE/1 -> LSM/12
  RFM_LEFT_LANE/1 -> LSM/13
  RFM_CURRENT_LANE/1 -> LSM/14
  RFM_RIGHT_LANE/1 -> LSM/15
  RFM_INTERSEC_ALERT/1 -> LSM/16
  RFM_BRANCH/1 -> LSM/17
  RFM_REC_LANES/1 -> LSM/18
  RFM_LINE_L1/1 -> LSM/19
  RFM_LINE_R1/1 -> LSM/20
  RFM_LINE_L2/1 -> LSM/21
  RFM_LINE_R2/1 -> LSM/22
  RFM_LINE_L3/1 -> LSM/23
  RFM_LINE_R3/1 -> LSM/24
  RFM_LINE_CL/1 -> LSM/25
  RFM_LINE_LB/1 -> LSM/26
  RFM_LINE_RB/1 -> LSM/27
  RFM_LINE_PRED/1 -> LSM/28
  RFM_LINEF_LB/1 -> LSM/29
  RFM_LINEF_RB/1 -> LSM/30
  RFM_LINE_ENTRY_CL/1 -> LSM/31
  RFM_LINE_EXIT_CL/1 -> LSM/32
  RFM_TSR/1 -> LSM/33
  VSM_ReqMRC/1 -> Terminator/1
  LSM/12 -> LSM_TJALineSource/1

== system Noa_Nofusion_angle/LPV/VSM ==
  VSM_VCAN_ECM : Inport  OutDataTypeStr=Bus: VCAN_ECM_MSG_BUS  PortDimensions=1  BusOutputAsStruct=on
  VSM_VCAN_DCT : Inport  Port=2  OutDataTypeStr=Bus: VCAN_DCT_MSG_BUS  PortDimensions=1  BusOutputAsStruct=on
  VSM_VCAN_HCU : Inport  Port=3  OutDataTypeStr=Bus: VCAN_HCU_MSG_BUS  PortDimensions=1  BusOutputAsStruct=on
  VSM_VCAN_ESP : Inport  Port=4  OutDataTypeStr=Bus: VCAN_ESP_MSG_BUS  PortDimensions=1  BusOutputAsStruct=on
  VSM_VCAN_EPS : Inport  Port=5  OutDataTypeStr=Bus: VCAN_EPS_MSG_BUS  PortDimensions=1  BusOutputAsStruct=on
  VSM_VCAN_PEPS : Inport  Port=6  OutDataTypeStr=Bus: VCAN_PEPS_MSG_BUS  PortDimensions=1  BusOutputAsStruct=on
  VSM_VCAN_BCM : Inport  Port=7  OutDataTypeStr=Bus: VCAN_BCM_MSG_BUS  PortDimensions=1  BusOutputAsStruct=on
  VSM_ACAmbTemp : Inport  Port=8  OutDataTypeStr=Bus: VCAN_AC_MSG_BUS  PortDimensions=1  BusOutputAsStruct=on
  VSM_VCAN_PBOX : Inport  Port=9  OutDataTypeStr=Bus: VCAN_PBOX_MSG_BUS  PortDimensions=1  BusOutputAsStruct=on
  VSM_VCAN_CSA : Inport  Port=10  OutDataTypeStr=Bus: VCAN_CSA_MSG_BUS  PortDimensions=1  BusOutputAsStruct=on
  VSM_VCAN_ABM : Inport  Port=11  OutDataTypeStr=Bus: VCAN_ABM_MSG_BUS  PortDimensions=1  BusOutputAsStruct=on
  VSM_VCAN_IP : Inport  Port=12  OutDataTypeStr=Bus: VCAN_IP_MSG_BUS  PortDimensions=1  BusOutputAsStruct=on
  VSM_VCAN_HUT : Inport  Port=13  OutDataTypeStr=Bus: VCAN_HUT_MSG_BUS  PortDimensions=1  BusOutputAsStruct=on
  VSM_VCAN_CR : Inport  Port=14  OutDataTypeStr=Bus: VCAN_CR_MSG_BUS  PortDimensions=1  BusOutputAsStruct=on
  VSM_VCAN_HC : Inport  Port=15  OutDataTypeStr=Bus: VCAN_HC_MSG_BUS  PortDimensions=1  BusOutputAsStruct=on
  VSM_VCAN_HAP : Inport  Port=16  OutDataTypeStr=Bus: VCAN_HAP_MSG_BUS  PortDimensions=1  BusOutputAsStruct=on
  DriverSts : Inport  Port=17  OutDataTypeStr=uint8  PortDimensions=1  BusOutputAsStruct=on
  CAL_VSM_CONFIG : Inport  Port=18  OutDataTypeStr=Bus: CAL_VSM_CONFIG_BUS  PortDimensions=1  BusOutputAsStruct=on
  DFIM_VSM_STS : Inport  Port=19  OutDataTypeStr=Bus: DFIM_VSM_STS_BUS  PortDimensions=1  BusOutputAsStruct=on
  RFM_LINE_L1 : Inport  Port=20  OutDataTypeStr=Bus: RFM_LINE_BUS  PortDimensions=1  BusOutputAsStruct=on
  RFM_LINE_R1 : Inport  Port=21  OutDataTypeStr=Bus: RFM_LINE_BUS  PortDimensions=1  BusOutputAsStruct=on
  RFM_LINE_LB : Inport  Port=22  OutDataTypeStr=Bus: RFM_LINE_BUS  PortDimensions=1  BusOutputAsStruct=on
  RFM_LINE_RB : Inport  Port=23  OutDataTypeStr=Bus: RFM_LINE_BUS  PortDimensions=1  BusOutputAsStruct=on
  LSM_UpdateCnt : Inport  Port=24  OutDataTypeStr=uint32  PortDimensions=1  BusOutputAsStruct=on
  LSM_TJA_ICA : Inport  Port=25  OutDataTypeStr=Bus: LSM_TJA_ICA_BUS  PortDimensions=1  BusOutputAsStruct=on
  LSM_HWA : Inport  Port=26  OutDataTypeStr=Bus: LSM_HWA_BUS  PortDimensions=1  BusOutputAsStruct=on
  LSM_LCK : Inport  Port=27  OutDataTypeStr=Bus: LSM_LCK_BUS  PortDimensions=1  BusOutputAsStruct=on
  LSM_ESS : Inport  Port=28  OutDataTypeStr=Bus: LSM_ESS_BUS  PortDimensions=1  BusOutputAsStruct=on
  TOS_ACCP0 : Inport  Port=29  OutDataTypeStr=Bus: TOS_ACCP0_BUS  PortDimensions=1  BusOutputAsStruct=on
  TOS_AEB_LONOBJ : Inport  Port=30  OutDataTypeStr=Bus: TOS_AEB_LONOBJ_BUS  PortDimensions=1  BusOutputAsStruct=on
  TOS_ELK : Inport  Port=31  OutDataTypeStr=Bus: TOS_ELK_BUS  PortDimensions=1  BusOutputAsStruct=on
  TOS_LCKIE : Inport  Port=32  OutDataTypeStr=Bus: TOS_LCKIE_BUS  PortDimensions=1  BusOutputAsStruct=on
  EHRV2_ROAD_INFO : Inport  Port=33  OutDataTypeStr=Bus: EHRV2_ROAD_INFO_BUS  PortDimensions=1  BusOutputAsStruct=on
  RFM_ROAD : Inport  Port=34  OutDataTypeStr=Bus: RFM_ROAD_BUS  PortDimensions=1  BusOutputAsStruct=on
  RFM_INTERSEC_ALERT : Inport  Port=35  OutDataTypeStr=Bus: RFM_INTERSEC_ALERT_BUS  PortDimensions=1  BusOutputAsStruct=on
  EHRV2_HutHandshake : Inport  Port=36  OutDataTypeStr=uint8  PortDimensions=1  BusOutputAsStruct=on
  EHRV2_HDR : Inport  Port=37  OutDataTypeStr=Bus: EHRV2_HDR_BUS  PortDimensions=1  BusOutputAsStruct=on
  axvRefMs2 : Inport  Port=38  OutDataTypeStr=single  PortDimensions=1  BusOutputAsStruct=on
  vxvRefMs : Inport  Port=39  OutDataTypeStr=single  PortDimensions=1  BusOutputAsStruct=on
  axvRoadSlopeMs2 : Inport  Port=40  OutDataTypeStr=single  PortDimensions=1  BusOutputAsStruct=on
  psiDtOpt : Inport  Port=41  OutDataTypeStr=single  PortDimensions=1  BusOutputAsStruct=on
  ayvRefMs2 : Inport  Port=42  OutDataTypeStr=single  PortDimensions=1  BusOutputAsStruct=on
  kapTraj : Inport  Port=43  OutDataTypeStr=single  PortDimensions=1  BusOutputAsStruct=on
  AEB_IPHUT_INFO : Inport  Port=44  OutDataTypeStr=Bus: AEB_IPHUT_INFO_BUS  PortDimensions=1  BusOutputAsStruct=on
  AEB_BRK_INFO : Inport  Port=45  OutDataTypeStr=Bus: AEB_BRK_INFO_BUS  PortDimensions=1  BusOutputAsStruct=on
  RFM_TSR : Inport  Port=46  OutDataTypeStr=Bus: RFM_TSR_BUS  PortDimensions=1  BusOutputAsStruct=on
  LATC_IFCTrqOvlCmdReqValue : Inport  Port=47  OutDataTypeStr=single  PortDimensions=1  BusOutputAsStruct=on
  LATC_IFCFuncTrqCmdReqFlag : Inport  Port=48  OutDataTypeStr=uint8  PortDimensions=1  BusOutputAsStruct=on
  VSM_TSR_INIT : Inport  Port=49  OutDataTypeStr=Bus: VSM_TSR_INIT_BUS  PortDimensions=1  BusOutputAsStruct=on
  PLAN_ACCPLAN : Inport  Port=50  OutDataTypeStr=Bus: PLAN_ACCPLAN_BUS  PortDimensions=1  BusOutputAsStruct=on
  PLAN_DriverOffConditionFulfilled : Inport  Port=51  OutDataTypeStr=boolean  PortDimensions=1  BusOutputAsStruct=on
  LSM_PilotSts : Inport  Port=52  OutDataTypeStr=uint8  PortDimensions=1  BusOutputAsStruct=on
  PLAN_ALC_Decision : Inport  Port=53  OutDataTypeStr=Bus: PLAN_ALC_DECS_BUS
  PLAN_DPC_ESS : Inport  Port=54  OutDataTypeStr=Bus: PLAN_DPC_ESS_BUS
  PLAN_NOH_SetSpdAdjReq : Inport  Port=55  OutDataTypeStr=boolean
  PLAN_NOH_SetSpdAdjVal : Inport  Port=56  OutDataTypeStr=uint8
  LSM_TJALineSource : Inport  Port=57
  Constant : Constant  Value=0  OutDataTypeStr=uint8
  VSM : ModelReference  ModelNameDialog=PubIfStateVSM_MDL.slx  SimulationMode=Normal  ModelReferenceVersion=1.109
  VSM_LON_CTRL : Outport  OutDataTypeStr=Bus: VSM_LON_CTRL_BUS  PortDimensions=1  BusOutputAsStruct=on
  VSM_LAT_CTRL : Outport  Port=2  OutDataTypeStr=Bus: VSM_LAT_CTRL_BUS  BusOutputAsStruct=on
  VSM_HMI : Outport  Port=3  OutDataTypeStr=Bus: VSM_HMI_BUS  PortDimensions=1  BusOutputAsStruct=on
  VSM_CTRL_LINE : Outport  Port=4  OutDataTypeStr=Bus: VSM_CTRL_LINE_BUS  PortDimensions=1  BusOutputAsStruct=on
  VSM_TSR : Outport  Port=5  OutDataTypeStr=Bus: VSM_TSR_BUS  PortDimensions=1  BusOutputAsStruct=on
  VSM_TSR_REMAIN : Outport  Port=6  OutDataTypeStr=Bus: VSM_TSR_REMAIN_BUS  BusOutputAsStruct=on
  VSM_UOM_LC : Outport  Port=7  OutDataTypeStr=Bus: VSM_UOM_LC_BUS
  DataCLCT : Outport  Port=8
  VSM_MRCReq : Outport  Port=9  OutDataTypeStr=uint8
  wires:
  VSM/6 -> VSM_TSR_REMAIN/1
  VSM/1 -> VSM_LON_CTRL/1
  VSM/2 -> VSM_LAT_CTRL/1
  VSM/4 -> VSM_CTRL_LINE/1
  VSM/5 -> VSM_TSR/1
  VSM/3 -> VSM_HMI/1
  VSM/8 -> DataCLCT/1
  VSM/7 -> VSM_UOM_LC/1
  VSM_VCAN_ECM/1 -> VSM/1
  VSM_VCAN_DCT/1 -> VSM/2
  VSM_VCAN_HCU/1 -> VSM/3
  VSM_VCAN_ESP/1 -> VSM/4
  VSM_VCAN_EPS/1 -> VSM/5
  VSM_VCAN_PEPS/1 -> VSM/6
  VSM_VCAN_BCM/1 -> VSM/7
  VSM_ACAmbTemp/1 -> VSM/8
  VSM_VCAN_PBOX/1 -> VSM/9
  VSM_VCAN_CSA/1 -> VSM/10
  VSM_VCAN_ABM/1 -> VSM/11
  VSM_VCAN_IP/1 -> VSM/12
  VSM_VCAN_HUT/1 -> VSM/13
  VSM_VCAN_CR/1 -> VSM/14
  VSM_VCAN_HC/1 -> VSM/15
  VSM_VCAN_HAP/1 -> VSM/16
  DriverSts/1 -> VSM/17
  CAL_VSM_CONFIG/1 -> VSM/18
  DFIM_VSM_STS/1 -> VSM/19
  RFM_LINE_L1/1 -> VSM/20
  RFM_LINE_R1/1 -> VSM/21
  RFM_LINE_LB/1 -> VSM/22
  RFM_LINE_RB/1 -> VSM/23
  LSM_UpdateCnt/1 -> VSM/24
  LSM_TJA_ICA/1 -> VSM/25
  LSM_HWA/1 -> VSM/26
  LSM_LCK/1 -> VSM/27
  LSM_ESS/1 -> VSM/28
  TOS_ACCP0/1 -> VSM/29
  TOS_AEB_LONOBJ/1 -> VSM/30
  TOS_ELK/1 -> VSM/31
  TOS_LCKIE/1 -> VSM/32
  EHRV2_ROAD_INFO/1 -> VSM/33
  RFM_ROAD/1 -> VSM/34
  RFM_INTERSEC_ALERT/1 -> VSM/35
  EHRV2_HutHandshake/1 -> VSM/36
  EHRV2_HDR/1 -> VSM/37
  axvRefMs2/1 -> VSM/38
  vxvRefMs/1 -> VSM/39
  axvRoadSlopeMs2/1 -> VSM/40
  psiDtOpt/1 -> VSM/41
  ayvRefMs2/1 -> VSM/42
  kapTraj/1 -> VSM/43
  AEB_IPHUT_INFO/1 -> VSM/44
  AEB_BRK_INFO/1 -> VSM/45
  RFM_TSR/1 -> VSM/46
  LATC_IFCTrqOvlCmdReqValue/1 -> VSM/47
  LATC_IFCFuncTrqCmdReqFlag/1 -> VSM/48
  VSM_TSR_INIT/1 -> VSM/49
  PLAN_ACCPLAN/1 -> VSM/50
  PLAN_DriverOffConditionFulfilled/1 -> VSM/51
  LSM_PilotSts/1 -> VSM/52
  PLAN_ALC_Decision/1 -> VSM/53
  PLAN_DPC_ESS/1 -> VSM/54
  PLAN_NOH_SetSpdAdjReq/1 -> VSM/55
  PLAN_NOH_SetSpdAdjVal/1 -> VSM/56
  Constant/1 -> VSM_MRCReq/1  "MRCReq"
  LSM_TJALineSource/1 -> ?
